simulink model "Musicmask"  (R2023b)
settings: Solver=FixedStepAuto  StartTime=0.0  StopTime=inf  RelTol=1e-3
undefined symbols (not defined in the file): MaskingMusic1, MIC_SPL
libraries: androidaudiovideolib x3, androiduilib x1
settings Model: Creator=The MathWorks, Inc.  LastModifiedBy=hp
settings SolverCC: MaxZcPerStep=1
settings OptimizationCC: EnhancedBackFolding=on  PassReuseOutputArgsThreshold=0  MaxStackSize=64  OptimizeBlockOrder=speed  DifferentSizesBufferReuse=on  OptimizationCustomize=off
settings DebuggingCC: ParameterTunabilityLossMsg=error  UnconnectedInputMsg=warning  UnconnectedOutputMsg=warning  UnconnectedLineMsg=warning
settings HardwareCC: ProdBitPerPointer=32  ProdBitPerSizeT=32  ProdBitPerPtrDiffT=32  ProdLargestAtomicInteger=Long  ProdLargestAtomicFloat=Double  ProdWordSize=32  ProdHWDeviceType=ARM Compatible->ARM Cortex  UseEmbeddedCoderFeatures=off  UseSimulinkCoderFeatures=off
settings ModelReferenceCC: EnableRefExpFcnMdlSchedulingChecks=on
settings RTWCC: Description=Embedded Coder  SystemTargetFile=ert.tlc  HardwareBoard=Android Device  TLCOptions="-aInlineSetEventsForThisBaseRateFcn=TLC_FALSE -aSuppressMultiTaskScheduler=TLC_FALSE  -aRateBasedStepFcn=0"  TemplateMakefile=ert_default_tmf  RTWVerbose=off  Toolchain=Android SDK/NDK Tools  DLArmComputeVersion=19.05
settings CodeAppCC: ForceParamTrailComments=on  OperatorAnnotations=on
settings ERTTargetCC: ERTCustomFileBanners=off  SupportContinuousTime=on  SupportNonInlinedSFcns=on  RemoveResetFunc=off  ModelStepFunctionPrototypeControlCompliant=off

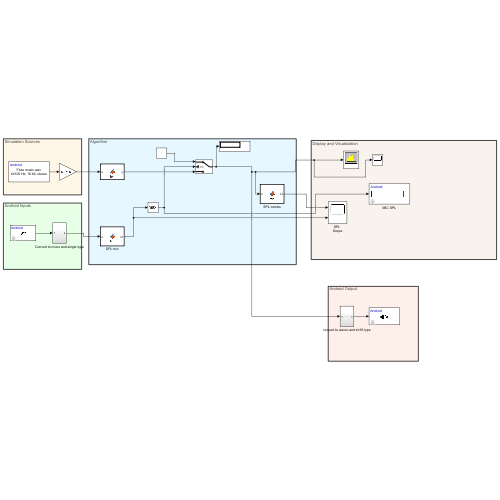
[thumbnail: Simulink's stored preview of the top-level diagram]
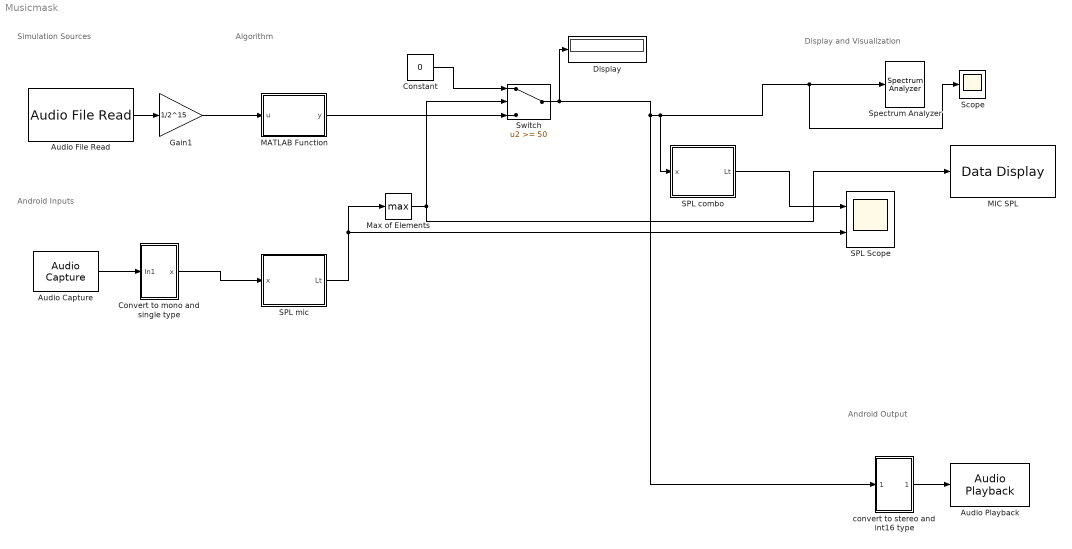
== system Musicmask ==
  note: Algorithm
  note: Android Inputs
  note: Android Output
  note: Display and Visualization
  note: Simulation Sources
  Audio Capture : androidaudiovideolib/Audio Capture  SampleFreq=44100  FrameSize=4410  SampleTime=0.1  SimulateUsing=Code generation  DeviceStr=0  QueueDuration=0  BlockPlatform=Android  AudioSamplingFreq=44100
  Audio File Read : androidaudiovideolib/Audio File Read  FileName=C:\Users\hp\Desktop\Flute music.wav  FrameSize=4410
  Audio Playback : androidaudiovideolib/Audio Playback  SampleFreq=44100  AudioSamplingFreq=44100  SampleTime=0.1  DeviceStr=0  QueueDuration=0  BlockPlatform=Android
  Constant : Constant  Value=0
  Convert to mono and single type : Subsystem
  Display : Display
  Gain1 : Gain  Gain=1/2^15  OutDataTypeStr=single
  MATLAB Function : MATLAB Function  TreatAsAtomicUnit=on
  MIC SPL : androiduilib/Data Display  DataDisplayId=MaskingMusic1/MIC_SPL  Format=Float  Precision=6  SimulateUsing=Code generation  blockPlatform=Android
  Max of Elements : MinMax  Function=max
  SPL Scope : Scope  NumInputPorts=2
  SPL combo : MATLAB Function  TreatAsAtomicUnit=on
  SPL mic : MATLAB Function  TreatAsAtomicUnit=on
  Scope : Scope
  Spectrum Analyzer : SpectrumAnalyzer  WindowPosition=[-4.000000,268.000000,800.000000,450.000000,]  ScopeFrameLocation=window  SampleRate=44100  Span=44100  StartFrequency=-22050  StopFrequency=22050  AveragingMethod=Exponential  YLimits=[-105.30043583,23.73250747]
  Switch : Switch  Threshold=50  SaturateOnIntegerOverflow=off  InputSameDT=off
  convert to stereo and int16 type : Subsystem
  wires:
  Audio Capture/1 -> Convert to mono and single type/1(In1)
  convert to stereo and int16 type/1(Out1) -> Audio Playback/1
  Audio File Read/1 -> Gain1/1
  SPL mic/1(Lt) -> SPL Scope/2, Max of Elements/1
  Convert to mono and single type/1(x) -> SPL mic/1(x)
  Max of Elements/1 -> Switch/2, MIC SPL/1
  Constant/1 -> Switch/1
  SPL combo/1(Lt) -> SPL Scope/1
  Switch/1 -> convert to stereo and int16 type/1(In1), SPL combo/1(x), Scope/1, Spectrum Analyzer/1, Display/1
  Gain1/1 -> MATLAB Function/1(u)
  MATLAB Function/1(y) -> Switch/3

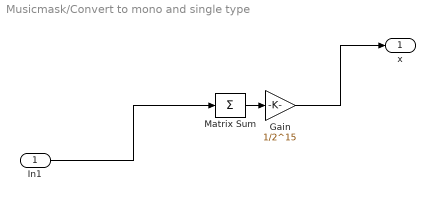
== system Musicmask/Convert to mono and single type ==
  In1 : Inport
  Gain : Gain  Gain=1/2^15  OutDataTypeStr=single
  Matrix Sum : Sum  Inputs=+  CollapseMode=Specified dimension  CollapseDim=2
  x : Outport
  wires:
  Matrix Sum/1 -> Gain/1
  Gain/1 -> x/1
  In1/1 -> Matrix Sum/1

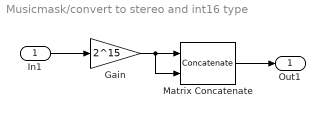
== system Musicmask/convert to stereo and int16 type ==
  In1 : Inport
  Gain : Gain  Gain=2^15  OutDataTypeStr=int16  SaturateOnIntegerOverflow=on
  Matrix Concatenate : Concatenate  Mode=Multidimensional array  ConcatenateDimension=2
  Out1 : Outport
  wires:
  In1/1 -> Gain/1
  Matrix Concatenate/1 -> Out1/1
  Gain/1 -> Matrix Concatenate/2, Matrix Concatenate/1

== matlab function Musicmask/SPL mic ==
  data: x input; Lt output
function Lt  = fcn(x)

SPL = splMeter(TimeWeighting="Fast", ...
    FrequencyWeighting="A-weighting", ...
    SampleRate=44100, ...
    TimeInterval=2);
% Lt = zeros(size(x)); 
% [Lt,Leq,Lpeak,Lmax] = SPL(x);

Lt= SPL(x);

== matlab function Musicmask/SPL combo ==
  data: x input; Lt output
function Lt  = fcn(x)

SPL = splMeter(TimeWeighting="Fast", ...
    FrequencyWeighting="A-weighting", ...
    SampleRate=44100, ...
    TimeInterval=10);
% Lt = zeros(size(x)); 
% [Lt,Leq,Lpeak,Lmax] = SPL(x);

Lt= SPL(x);

== matlab function Musicmask/MATLAB Function ==
  data: u input; y output
function y = fcn(u)

y = u(:,1);
